simulink subsystem "deg2TimeDelay"  (R2024a)
settings: Solver=VariableStepAuto  StartTime=0.0  StopTime=10.0  RelTol=1e-3
settings Model: Creator=Admin  LastModifiedBy=Admin

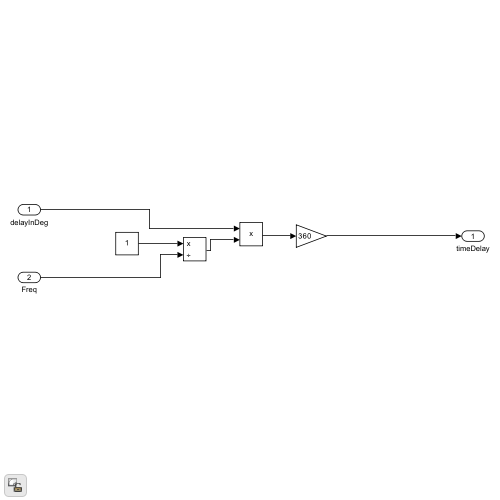
[thumbnail: Simulink's stored preview of the top-level diagram]
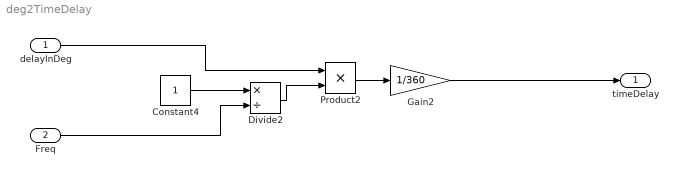
== system deg2TimeDelay ==
  delayInDeg : Inport
  Freq : Inport  Port=2
  Constant4 : Constant
  Divide2 : Product  Inputs=*/
  Gain2 : Gain  Gain=1/360
  Product2 : Product
  timeDelay : Outport
  wires:
  Divide2/1 -> Product2/2
  Constant4/1 -> Divide2/1
  Product2/1 -> Gain2/1
  Gain2/1 -> timeDelay/1
  delayInDeg/1 -> Product2/1
  Freq/1 -> Divide2/2
